simulink model "mpc_wbc_CONTROL"  (R2018a)
settings: Solver=VariableStepAuto  StartTime=0.0  StopTime=100.0  RelTol=1e-3
undefined symbols (not defined in the file or in its folder): D_d, dragcoeff, G_d, M_d, pos_init, pp, quat_init, snake, x_init
libraries: dspindex x1
settings Model: Creator=sarava  LastModifiedBy=12037

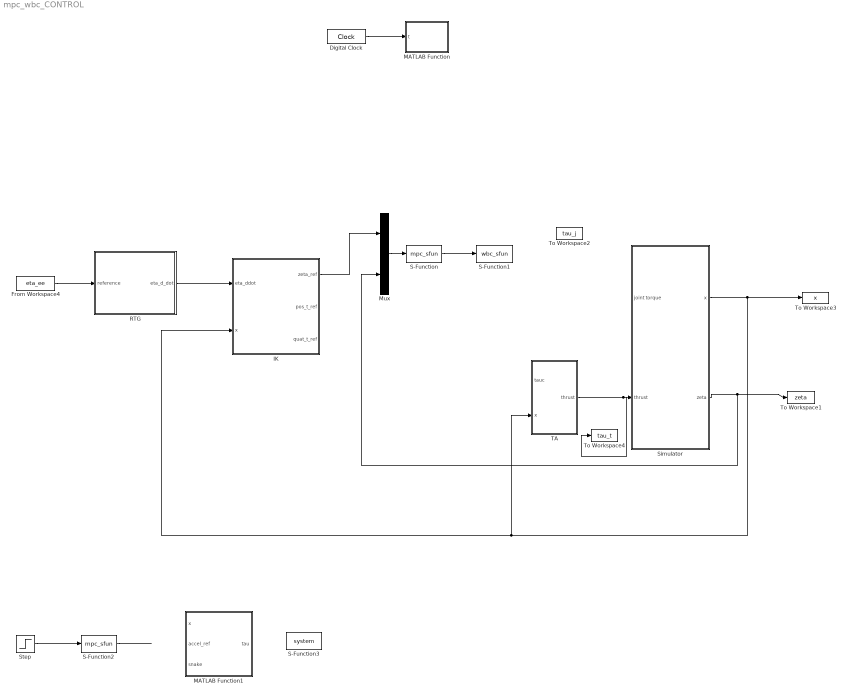
== system mpc_wbc_CONTROL ==
  Digital Clock : DigitalClock
  From Workspace4 : FromWorkspace  VariableName=eta_ee  SampleTime=0
  IK : Subsystem
  MATLAB Function : MATLAB Function  TreatAsAtomicUnit=on
  MATLAB Function1 : MATLAB Function  TreatAsAtomicUnit=on
  Mux : Mux  Inputs=2
  RTG : Subsystem
  S-Function : S-Function  FunctionName=mpc_sfun  SFunctionDeploymentMode=off  EnableBusSupport=off
  S-Function1 : S-Function  FunctionName=wbc_sfun  SFunctionDeploymentMode=off  EnableBusSupport=off
  S-Function2 : S-Function  FunctionName=mpc_sfun  SFunctionDeploymentMode=off  EnableBusSupport=off
  S-Function3 : S-Function  SFunctionDeploymentMode=off  EnableBusSupport=off
  Simulator : Subsystem
  Step : Step  Time=2  After=0.5  SampleTime=0
  TA : Subsystem
  To Workspace1 : ToWorkspace  VariableName=zeta  SaveFormat=Timeseries  SampleTime=-1
  To Workspace2 : ToWorkspace  VariableName=tau_j  SaveFormat=Timeseries  SampleTime=-1
  To Workspace3 : ToWorkspace  VariableName=x  SaveFormat=Timeseries  SampleTime=-1
  To Workspace4 : ToWorkspace  VariableName=tau_t  SaveFormat=Timeseries  SampleTime=-1
  wires:
  Digital Clock/1 -> MATLAB Function/1(t)
  Simulator/2(zeta) -> Mux/2, To Workspace1/1
  Simulator/1(x) -> IK/2(x), TA/2("x "), To Workspace3/1
  From Workspace4/1 -> RTG/1(reference)
  RTG/1(eta_d_dot) -> IK/1(eta_ddot)
  ? -> To Workspace2/1, Simulator/1(joint torque)
  TA/1(thrust) -> To Workspace4/1, Simulator/2(thrust)
  Mux/1 -> S-Function/1
  IK/1(zeta_ref) -> Mux/1
  S-Function/1 -> S-Function1/1
  S-Function2/1 -> ?
  Step/1 -> S-Function2/1

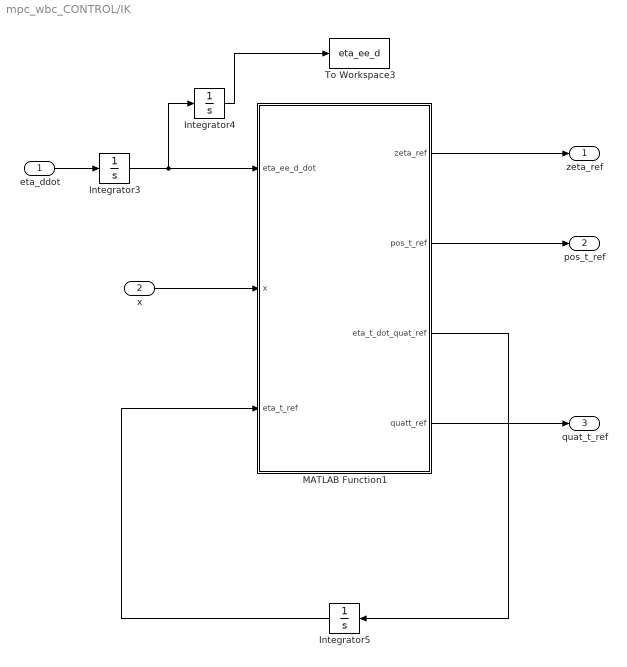
== system mpc_wbc_CONTROL/IK ==
  eta_ddot : Inport
  x : Inport  Port=2
  Integrator3 : Integrator
  Integrator4 : Integrator
  Integrator5 : Integrator  InitialCondition=[pos_init quat_init]'
  MATLAB Function1 : MATLAB Function  TreatAsAtomicUnit=on
  To Workspace3 : ToWorkspace  VariableName=eta_ee_d  SaveFormat=Timeseries  SampleTime=-1
  zeta_ref : Outport
  pos_t_ref : Outport  Port=2
  quat_t_ref : Outport  Port=3
  wires:
  MATLAB Function1/1(zeta_ref) -> zeta_ref/1
  x/1 -> MATLAB Function1/2(x)
  MATLAB Function1/2(pos_t_ref) -> pos_t_ref/1
  MATLAB Function1/3(eta_t_dot_quat_ref) -> Integrator5/1
  Integrator4/1 -> To Workspace3/1
  Integrator5/1 -> MATLAB Function1/3(eta_t_ref)
  MATLAB Function1/4(quatt_ref) -> quat_t_ref/1
  eta_ddot/1 -> Integrator3/1
  Integrator3/1 -> Integrator4/1, MATLAB Function1/1(eta_ee_d_dot)

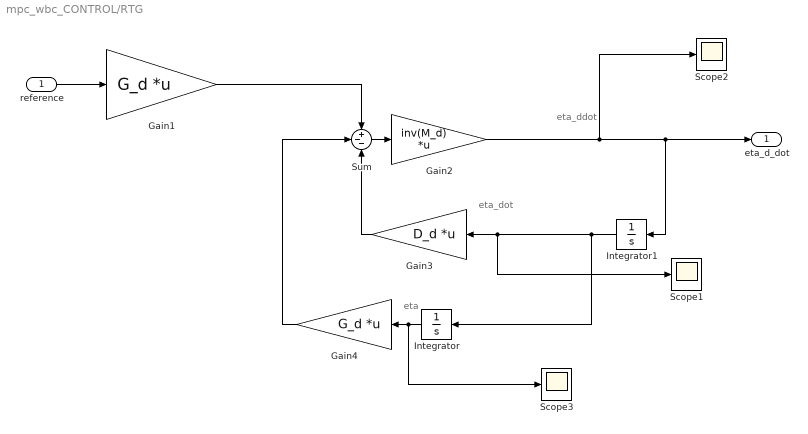
== system mpc_wbc_CONTROL/RTG ==
  note: eta_dot
  note: eta
  note: eta_ddot
  reference : Inport
  Gain1 : Gain  Gain=G_d  Multiplication=Matrix(K*u) (u vector)
  Gain2 : Gain  Gain=inv(M_d)  Multiplication=Matrix(K*u) (u vector)
  Gain3 : Gain  Gain=D_d  Multiplication=Matrix(K*u) (u vector)
  Gain4 : Gain  Gain=G_d  Multiplication=Matrix(K*u) (u vector)
  Integrator : Integrator
  Integrator1 : Integrator
  Scope1 : Scope
  Scope2 : Scope
  Scope3 : Scope
  Sum : Sum  Inputs=+--
  eta_d_dot : Outport
  wires:
  Gain2/1 -> Scope2/1, eta_d_dot/1, Integrator1/1
  Gain1/1 -> Sum/1
  Sum/1 -> Gain2/1
  reference/1 -> Gain1/1
  Integrator1/1 -> Integrator/1, Scope1/1, Gain3/1
  Integrator/1 -> Scope3/1, Gain4/1
  Gain3/1 -> Sum/3
  Gain4/1 -> Sum/2

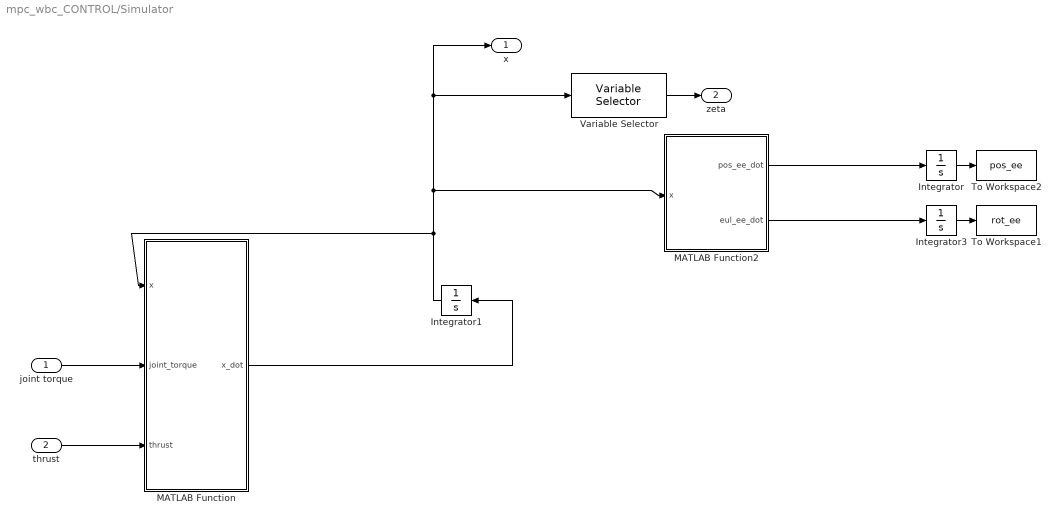
== system mpc_wbc_CONTROL/Simulator ==
  joint torque : Inport
  thrust : Inport  Port=2
  Integrator : Integrator
  Integrator1 : Integrator  InitialCondition=x_init
  Integrator3 : Integrator
  MATLAB Function : MATLAB Function  TreatAsAtomicUnit=on
  MATLAB Function2 : MATLAB Function  TreatAsAtomicUnit=on
  To Workspace1 : ToWorkspace  VariableName=rot_ee  SaveFormat=Timeseries  SampleTime=-1
  To Workspace2 : ToWorkspace  VariableName=pos_ee  SaveFormat=Timeseries  SampleTime=-1
  Variable Selector : dspindex/Variable Selector  NumInputs=1  rowsOrCols=Rows  IdxMode=Fixed  Elements=16:29  ZerOneIdxMode=One-based  errmode=Clip Index  FillMode=on  FillValues=0
  x : Outport
  zeta : Outport  Port=2
  wires:
  joint torque/1 -> MATLAB Function/2(joint_torque)
  thrust/1 -> MATLAB Function/3(thrust)
  Variable Selector/1 -> zeta/1
  MATLAB Function/1(x_dot) -> Integrator1/1
  Integrator1/1 -> Variable Selector/1, x/1, MATLAB Function2/1(x), MATLAB Function/1(x)
  Integrator/1 -> To Workspace2/1
  MATLAB Function2/1(pos_ee_dot) -> Integrator/1
  MATLAB Function2/2(eul_ee_dot) -> Integrator3/1
  Integrator3/1 -> To Workspace1/1

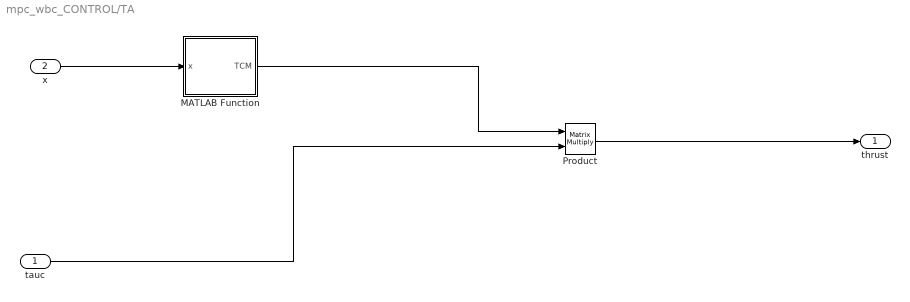
== system mpc_wbc_CONTROL/TA ==
  "tauc " : Inport
  "x " : Inport  Port=2
  MATLAB Function : MATLAB Function  TreatAsAtomicUnit=on
  Product : Product  Multiplication=Matrix(*)
  thrust : Outport
  wires:
  "x "/1 -> MATLAB Function/1(x)
  MATLAB Function/1(TCM) -> Product/1
  "tauc "/1 -> Product/2
  Product/1 -> thrust/1

== matlab function mpc_wbc_CONTROL/MATLAB Function1 ==
  data: x input; tau output; accel_ref input; snake input
function tau = wbc(x, accel_ref, snake)
% x: 状态（pos(3)+quat(4)+theta(8)+zeta(14)）
% accel_ref: MPC输出的关节加速度（8维）
theta = x(8:15); zeta = x(16:29);

% 计算惯性矩阵（调用slendermass.m）
M = slendermass(theta, snake);

% 科里奥利力和重力（调用comp_cdg.m）
[C,G] = comp_cdg(theta, zeta, snake);

% 关节力矩计算
tau = M*accel_ref + C*zeta + G;

% 力矩限幅（±50N·m）
tau = max(min(tau, 50), -50);

== matlab function mpc_wbc_CONTROL/Simulator/MATLAB Function ==
  data: x input; x_dot output; joint_torque input; thrust input; pp parameter; snake parameter; dragcoeff parameter
function x_dot  = dyn(x,joint_torque,thrust , pp, snake, dragcoeff)

pos       =  x(1:3);
quat      =  x(4:7);
theta     =  x(8 : 6+snake.n);
zeta      =  x(7+snake.n : 11+2*snake.n);
%Compute rotation matrices and jacobians
[Rcdg,Jcdg]=comp_rot_jac_mcdg(quat,theta,snake);
%Compute mass matrix
M         =  comp_mass(Jcdg,snake);

%Compute relative velocity to take into account the effect of current
velc_h    =  Rcdg(:,:,1)'*pp.velc;
nu        =  zeta(1:6);
zeta(1:3) =  zeta(1:3)-velc_h;

%Compute coriolis, drag, and hydrostatic terms with the relative velocity
[c, d, g] =  comp_cdg(Jcdg,Rcdg,theta,snake,pp,dragcoeff,zeta);
%Compute the thrust-configuration matrix
B         =  comp_TCM(Jcdg,snake);


%Compute the relative acceleration
zeta_dot      =  M\([B [zeros(6,8); eye(8)]]*[thrust;joint_torque]-c-d-g);% -c-d-g

%Remove the effect of current
zeta_dot(1:3) = zeta_dot(1:3)-cross(nu(4:6),velc_h);
%Compute the time derivatives of position and orientation
pos_dot   =  Rcdg(:,:,1)*nu(1:3);  
quat_dot  =  TransAngQ(quat)*nu(4:6)+1*(1-quat'*quat)*quat; 
%Assemble derivative of the state vector
x_dot = [pos_dot ; quat_dot ; zeta(7:snake.n+5) ; zeta_dot];
end

== matlab function mpc_wbc_CONTROL/MATLAB Function ==
  data: t input
function fcn(t)
%#codegen
coder.extrinsic('fprintf');
persistent firstTime

if isempty(firstTime)
    firstTime = false;
    fprintf('Starting Now\n');
end

fprintf('time = %.4f\n',t);

== matlab function mpc_wbc_CONTROL/TA/MATLAB Function ==
  data: TCM output; x input; snake parameter
function TCM = fcn(x , snake)
quat      =  x(4:7);
theta     =  x(8 : 6+snake.n);
[~, J]    =  comp_rot_jac(quat,theta,snake);
B        =  comp_TCM(J,snake);
TCM_t=B(1:6,:);
TCM=transpose(TCM_t)/(TCM_t*transpose(TCM_t));

== matlab function mpc_wbc_CONTROL/Simulator/MATLAB Function2 ==
  data: pos_ee_dot output; x input; snake parameter; eul_ee_dot output
function [pos_ee_dot, eul_ee_dot] = snake2points(x,snake)
   quat         = x(4:7);
   theta        = x(8 : 6+snake.n);
    zeta      =  x(7+snake.n : 11+2*snake.n);

   [R,J]=comp_rot_jac(quat,theta,snake);
  
   eul_ee=rotm2eul(R(:,:,10), 'XYZ')';
   Jinv=Jinv_fromeul(eul_ee);
   eta_ee_dot=[R(:,:,10) zeros(3); zeros(3) Jinv]*J(:,:,10)*zeta;
   x_ee_dot=[R(:,:,10) zeros(3); zeros(3) R(:,:,10)]*J(:,:,10)*zeta;
   pos_ee_dot=x_ee_dot(1:3);
   omega_ee=x_ee_dot(4:6);
   eul_ee_dot=eta_ee_dot(4:6);
end

== matlab function mpc_wbc_CONTROL/IK/MATLAB Function1 ==
  data: eta_ee_d_dot input; x input; eta_t_ref input; zeta_ref output; snake parameter; pos_t_ref output; eta_t_dot_quat_ref output; quatt_ref output
function [zeta_ref , pos_t_ref,eta_t_dot_quat_ref, quatt_ref] = fucn(eta_ee_d_dot,x,eta_t_ref, snake)
quat      =  x(4:7);
theta     =  x(8 : 6+snake.n);
[R, J_t]    =  comp_rot_jac(quat,theta,snake);


eul_ee=rotm2eul(R(:,:,10), 'XYZ')';

Jinv=Jinv_fromeul(eul_ee);
J=[R(:,:,10) zeros(3); zeros(3) Jinv]*J_t(:,:,10);

zeta_ref=J'/(J*J'+0.0001*eye(6))*(eta_ee_d_dot);%+K*sigma_tilde);
eta_ee_ref_dot=J*zeta_ref;



quatt_ref=eta_t_ref(4:7);
pos_t_ref=eta_t_ref(1:3);
R_tail=quat2rotm(quatt_ref');

pos_t_dot   =  R_tail(:,:,1)*zeta_ref(1:3);  
quat_t_dot  =  TransAngQ(quatt_ref)*zeta_ref(4:6)+1*(1-quatt_ref'*quatt_ref)*quatt_ref; ruh

eta_t_dot_quat_ref=[pos_t_dot; quat_t_dot];
end
